simulink model "sampleModel1992"  (R2023a)
settings: Solver=VariableStepAuto  StartTime=0.0  StopTime=10.0  RelTol=1e-3
libraries: simulink x3, hdlsllib x2
settings Model: Creator=user1  LastModifiedBy=user1

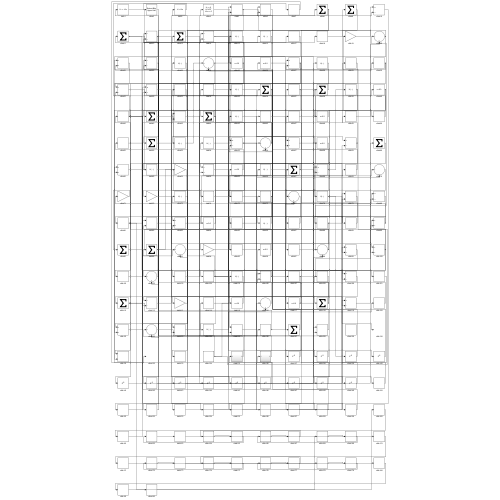
[thumbnail: Simulink's stored preview of the top-level diagram]
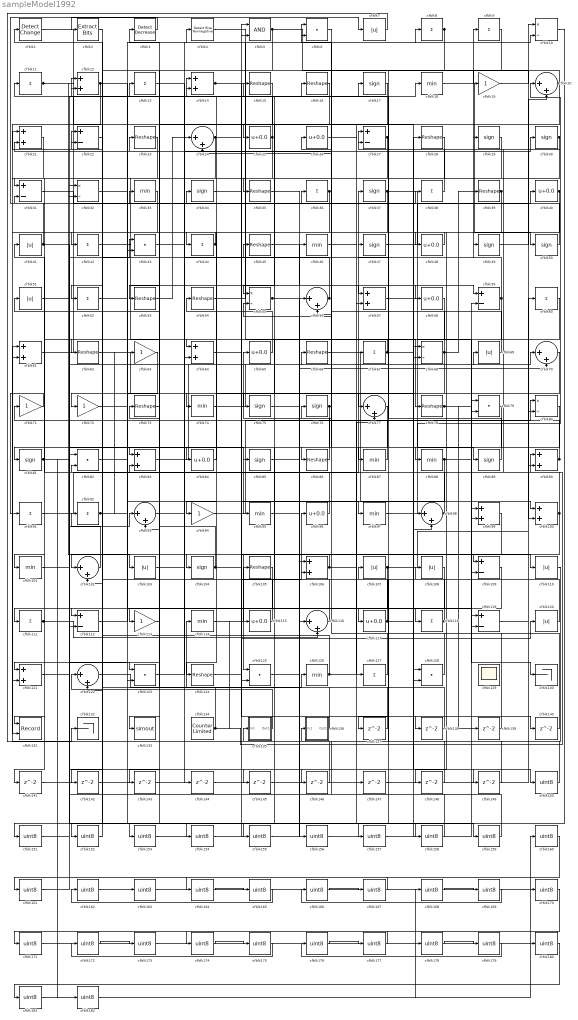
== system sampleModel1992 ==
  cfblk1 : simulink/Logic and Bit Operations/Detect Change  vinit=0  OutDataTypeStr=boolean
      settings: LibrarySourceBlock=|
      | hdlsllib/Logic and Bit
      | Operations/Detect
      | Change
  cfblk{10,32,55,68,80} (5 alike) : Product  Inputs=*/  RndMeth=Zero  SaturateOnIntegerOverflow=on
  cfblk{12,14,21,57,61,64,83,90,99..100,106,121} (12 alike) : Sum
  cfblk{18,33,46,74,87..88,95,97,101,114,126} (11 alike) : MinMax
  cfblk{20,24,56,70,77,93,98,102,116,122} (10 alike) : Sum  Inputs=|++
  cfblk{7,41,51,69,103,107..108,110,120} (9 alike) : Abs  SaturateOnIntegerOverflow=off
  cfblk{17,29..30,34,37,47,49..50,75..76,81,85,89,104} (14 alike) : Signum
  cfblk{15..16,23,28,35,39,45,53..54,62,66,73,78,86,105,124} (16 alike) : Reshape
  cfblk{22,27,31,59,109,112,119} (7 alike) : Sum  Inputs=+-
  cfblk{8..9,11,13,36,38,42,44,52,60,67,91..92,111,118,127} (16 alike) : Sum  Inputs=+
  cfblk{19,63,71..72,94,113} (6 alike) : Gain
  cfblk{25..26,40,48,58,65,84,96,115,117} (10 alike) : Bias  Bias=0.0  SaturateOnIntegerOverflow=off
  cfblk{6,43,79,82,123,125,128} (7 alike) : DotProduct  OutDataTypeStr=Inherit: Inherit via internal rule
  cfblk129 : Scope
      settings: Floating=on
  cfblk130 : Terminator
  cfblk131 : Record  FileSettingsInternal="{\"entries\":[{\"content\":{\"excelSettings\":{\"content\":{},\"type\":\"Streamout.ExcelSettings\"}},\"type\":\"Streamout.FileSettingStorage\",\"uuid\":\"\"}],\"packageUris\":[\"http:\\/\\/schema.mathworks.com\\/mf0\\/streamout_blocks\\/R2020a\"],\"version\":\"1.0\"}"  Layout=[1 1]  SignalsInternal="{\"entries\":[{\"content\":{\"signals\":[{\"content\":{\"blockPath\":[],\"dimensions\":[1],\"domain\":\"\",\"lineColor\":\"#a2142f\",\"plots\":[1],\"port\":1,\"signalID\":5711,\"signalName\":\"XY Graph:1\"},\"type\":\"RecordBlkView.Signal\",\"uuid\":\"\"},{\"content\":{\"blockPath\":[],\"dimensions\":[1],\"domain\":\"\",\"lineColor\":\"#139fff\",\"plots\":[1],\"port\":2,\"signalID\":5714,\"signalName\":\"XY Graph:2\"},\"type\":\"RecordBlkView.Signal\",\"uuid\":\"\"}]},\"type\":\"RecordBlkView.InputSignals\",\"uuid\":\"\"}],\"packageUris\":[\"http:\\/\\/schema.mathworks.com\\/mf0\\/streamout_blocks\\/R2020a\"],\"version\":\"1.0\"}"  VisualizationBindings="{\"xyplotplugin\":{\"info\":[{\"series\":[{\"bindingParametersList\":[{\"parameter\":\"X-Axis\",\"signalID\":5711,\"signalName\":\"XY Graph:1\"},{\"parameter\":\"Y-Axis\",\"signalID\":5714,\"signalName\":\"XY Graph:2\"}],\"seriesID\":43094}],\"subplotID\":1}]}}"  CompatibilityTag=XY  st=-1
  cfblk132 : Terminator
  cfblk133 : ToWorkspace  VariableName=simout  SaveFormat=Timeseries  SampleTime=-1
  cfblk134 : hdlsllib/Sources/Counter Limited  uplimit=7  tsamp=-1
  cfblk135 : Subsystem
      settings: LibrarySourceBlock=|
      | hdlsllib/Ports &
      | Subsystems/Subsystem
  cfblk136 : Subsystem
      settings: LibrarySourceBlock=|
      | hdlsllib/Ports &
      | Subsystems/Subsystem
  cfblk{137..149} (13 alike) : Delay  SampleTime=1
  cfblk{150..182} (33 alike) : DataTypeConversion  OutDataTypeStr=uint8  SaturateOnIntegerOverflow=off  RndMeth=Floor
  cfblk2 : simulink/Logic and Bit Operations/Extract Bits  bitsToExtract=Upper half  numBits=8  bitIdxRange=[0 7]  outScalingMode=Preserve fixed-point scaling
      settings: LibrarySourceBlock=|
      | hdlsllib/Logic and Bit
      | Operations/Extract Bits
  cfblk3 : simulink/Logic and Bit Operations/Detect Decrease  vinit=0.0  OutDataTypeStr=boolean
      settings: LibrarySourceBlock=|
      | hdlsllib/Logic and Bit
      | Operations/Detect
      | Decrease
  cfblk4 : hdlsllib/Logic and Bit Operations/Detect Rise Nonnegative  vinit=0  OutDataTypeStr=boolean
  cfblk5 : Logic  AllPortsSameDT=off  OutDataTypeStr=boolean
  wires:
  cfblk99/1 -> cfblk104/1
  cfblk53/1 -> cfblk24/1
  cfblk116/1 -> cfblk96/1
  cfblk56/1 -> cfblk13/1, cfblk22/2
  cfblk38/1 -> cfblk27/1
  cfblk94/1 -> cfblk80/1
  cfblk135/1(Out1) -> cfblk122/1
  cfblk86/1 -> cfblk65/1
  cfblk11/1 -> cfblk103/1, cfblk16/1
  cfblk63/1 -> cfblk72/1
  cfblk23/1 -> cfblk121/1
  cfblk25/1 -> cfblk11/1, cfblk121/2, cfblk81/1
  cfblk108/1 -> cfblk112/1
  cfblk109/1 -> cfblk113/1
  cfblk103/1 -> cfblk30/1
  cfblk113/1 -> cfblk33/1
  cfblk97/1 -> cfblk20/1
  cfblk106/1 -> cfblk102/1, cfblk109/1
  cfblk57/1 -> cfblk89/1
  cfblk136/1(Out1) -> cfblk114/1
  cfblk73/1 -> cfblk133/1
  cfblk4/1 -> cfblk78/1
  cfblk90/1 -> cfblk71/1, cfblk87/1
  cfblk66/1 -> cfblk100/1
  cfblk95/1 -> cfblk46/1
  cfblk117/1 -> cfblk12/1, cfblk149/1
  cfblk59/1 -> cfblk9/1, cfblk101/1
  cfblk50/1 -> cfblk3/1
  cfblk61/1 -> cfblk17/1
  cfblk41/1 -> cfblk7/1, cfblk123/2, cfblk85/1, cfblk154/1
  cfblk105/1 -> cfblk111/1
  cfblk20/1 -> cfblk19/1, cfblk137/1
  cfblk101/1 -> cfblk70/1
  cfblk70/1 -> cfblk124/1
  cfblk126/1 -> cfblk22/1, cfblk77/2
  cfblk77/1 -> cfblk83/1
  cfblk39/1 -> cfblk88/1, cfblk48/1
  cfblk55/1 -> cfblk58/1, cfblk138/1
  cfblk100/1 -> cfblk125/1, cfblk15/1, cfblk29/1, cfblk142/1
  cfblk8/1 -> cfblk123/1, cfblk157/1
  cfblk74/1 -> cfblk37/1
  cfblk18/1 -> cfblk50/1
  cfblk67/1 -> cfblk64/1, cfblk109/2
  cfblk29/1 -> cfblk122/2
  cfblk65/1 -> cfblk54/1
  cfblk119/1 -> cfblk60/1
  cfblk36/1 -> cfblk86/1, cfblk61/2
  cfblk122/1 -> cfblk126/1
  cfblk115/1 -> cfblk83/2
  cfblk71/1 -> cfblk91/1
  cfblk54/1 -> cfblk8/1
  cfblk120/1 -> cfblk76/1
  cfblk121/1 -> cfblk93/1
  cfblk89/1 -> cfblk14/1
  cfblk114/1 -> cfblk105/1
  cfblk2/1 -> cfblk102/2
  cfblk80/1 -> cfblk95/1
  cfblk47/1 -> cfblk40/1
  cfblk83/1 -> cfblk69/1
  cfblk27/1 -> cfblk35/1, cfblk64/2
  cfblk5/1 -> cfblk100/2, cfblk152/1
  cfblk21/1 -> cfblk31/1
  cfblk123/1 -> cfblk49/1
  cfblk91/1 -> cfblk67/1
  cfblk96/1 -> cfblk73/1
  cfblk9/1 -> cfblk53/1
  cfblk60/1 -> cfblk75/1
  cfblk16/1 -> cfblk55/1
  cfblk62/1 -> cfblk98/1
  cfblk42/1 -> cfblk59/1
  cfblk12/1 -> cfblk74/1, cfblk131/2
  cfblk17/1 -> cfblk25/1
  cfblk52/1 -> cfblk97/1
  cfblk102/1 -> cfblk92/1
  cfblk107/1 -> cfblk117/1, cfblk90/2
  cfblk72/1 -> cfblk118/1
  cfblk19/1 -> cfblk10/1
  cfblk76/1 -> cfblk131/1, cfblk6/1
  cfblk7/1 -> cfblk132/1
  cfblk40/1 -> cfblk84/1, cfblk148/1
  cfblk87/1 -> cfblk26/1
  cfblk88/1 -> cfblk59/2, cfblk125/2
  cfblk49/1 -> cfblk20/2
  cfblk111/1 -> cfblk116/2, cfblk14/2
  cfblk22/1 -> cfblk52/1
  cfblk24/1 -> cfblk18/1, cfblk62/1
  cfblk58/1 -> cfblk112/2
  cfblk44/1 -> cfblk94/1, cfblk42/1
  cfblk128/1 -> cfblk21/2
  cfblk124/1 -> cfblk120/1
  cfblk104/1 -> cfblk51/1, cfblk106/2, cfblk6/2, cfblk66/1
  cfblk98/1 -> cfblk41/1, cfblk12/2
  cfblk84/1 -> cfblk34/1
  cfblk125/1 -> cfblk106/1
  cfblk78/1 -> cfblk130/1, cfblk139/1
  cfblk6/1 -> cfblk56/2
  cfblk110/1 -> cfblk135/1(In1)
  cfblk34/1 -> cfblk119/2
  cfblk118/1 -> cfblk45/1, cfblk108/1
  cfblk127/1 -> cfblk55/2
  cfblk30/1 -> cfblk68/2, cfblk27/2
  cfblk64/1 -> cfblk110/1
  cfblk134/1 -> cfblk90/1, cfblk93/2, cfblk115/1
  cfblk112/1 -> cfblk4/1
  cfblk93/1 -> cfblk10/2
  cfblk14/1 -> cfblk127/1, cfblk140/1
  cfblk85/1 -> cfblk70/2
  cfblk81/1 -> cfblk43/1, cfblk182/1
  cfblk37/1 -> cfblk99/2, cfblk43/2
  cfblk1/1 -> cfblk128/2
  cfblk48/1 -> cfblk44/1
  cfblk69/1 -> cfblk23/1
  cfblk92/1 -> cfblk38/1, cfblk63/1
  cfblk31/1 -> cfblk36/1
  cfblk45/1 -> cfblk57/1
  cfblk35/1 -> cfblk57/2
  cfblk68/1 -> cfblk77/1, cfblk39/1, cfblk47/1
  cfblk3/1 -> cfblk2/1
  cfblk137/1 -> cfblk1/1
  cfblk138/1 -> cfblk21/1
  cfblk139/1 -> cfblk31/2
  cfblk140/1 -> cfblk24/2
  cfblk33/1 -> cfblk141/1
  cfblk141/1 -> cfblk98/2
  cfblk142/1 -> cfblk5/2
  cfblk15/1 -> cfblk143/1
  cfblk143/1 -> cfblk128/1
  cfblk13/1 -> cfblk144/1
  cfblk144/1 -> cfblk56/1
  cfblk51/1 -> cfblk145/1
  cfblk145/1 -> cfblk99/1
  cfblk43/1 -> cfblk146/1
  cfblk146/1 -> cfblk61/1
  cfblk46/1 -> cfblk147/1
  cfblk147/1 -> cfblk80/2
  cfblk148/1 -> cfblk68/1
  cfblk149/1 -> cfblk107/1
  cfblk82/1 -> cfblk150/1
  cfblk150/1 -> cfblk119/1
  cfblk10/1 -> cfblk151/1
  cfblk151/1 -> cfblk82/1
  cfblk152/1 -> cfblk82/2
  cfblk28/1 -> cfblk153/1
  cfblk153/1 -> cfblk5/1
  cfblk154/1 -> cfblk28/1
  cfblk79/1 -> cfblk155/1
  cfblk155/1 -> cfblk116/1
  cfblk75/1 -> cfblk156/1
  cfblk156/1 -> cfblk79/1
  cfblk157/1 -> cfblk79/2
  cfblk32/1 -> cfblk158/1
  cfblk158/1 -> cfblk136/1(In1)
  cfblk26/1 -> cfblk159/1
  cfblk159/1 -> cfblk32/1
  cfblk160/1 -> cfblk161/1
  cfblk161/1 -> cfblk32/2
  cfblk162/1 -> cfblk163/1
  cfblk163/1 -> cfblk160/1
  cfblk164/1 -> cfblk165/1
  cfblk165/1 -> cfblk162/1
  cfblk166/1 -> cfblk167/1
  cfblk167/1 -> cfblk164/1
  cfblk168/1 -> cfblk169/1
  cfblk169/1 -> cfblk166/1
  cfblk170/1 -> cfblk171/1
  cfblk171/1 -> cfblk168/1
  cfblk172/1 -> cfblk173/1
  cfblk173/1 -> cfblk170/1
  cfblk174/1 -> cfblk175/1
  cfblk175/1 -> cfblk172/1
  cfblk176/1 -> cfblk177/1
  cfblk177/1 -> cfblk174/1
  cfblk178/1 -> cfblk179/1
  cfblk179/1 -> cfblk176/1
  cfblk180/1 -> cfblk181/1
  cfblk181/1 -> cfblk178/1
  cfblk182/1 -> cfblk180/1

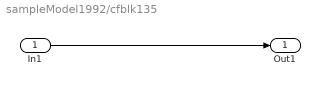
== system sampleModel1992/cfblk135 ==
  In1 : Inport
  Out1 : Outport
  wires:
  In1/1 -> Out1/1

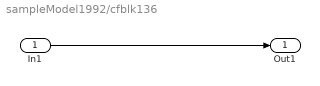
== system sampleModel1992/cfblk136 ==
  In1 : Inport
  Out1 : Outport
  wires:
  In1/1 -> Out1/1
